simulink subsystem "Shooter_Arm_Controls"  (R2023b)
settings: Solver=VariableStepAuto  StartTime=0.0  StopTime=10.0  RelTol=1e-3
undefined symbols (not defined in the file): Back_AA_Bot_Max_Ext, Back_AA_Bot_Min_Ext, Back_AA_length, Back_AA_spacing, Back_AA_Top_Max_Ext, Back_AA_Top_Min_Ext, Front_AA_length, Front_AA_Max_Ext, Front_AA_Min_Ext, Front_AA_spacing, l_1, l_10, l_11, l_2, l_3, l_4, l_5, l_6, l_7, l_8, l_9, Speaker_Angle_out, Speaker_Distance_in, Speaker_Distance_Offset, Speaker_Gap_out, Speaker_Height_out, TEST_Speaker_Angle, TEST_Speaker_Gap, TEST_Speaker_Height
libraries: Controls_Components_lib x5, simulink x4, simulink_need_slupdate x3
settings Model: Creator=ander  LastModifiedBy=ander

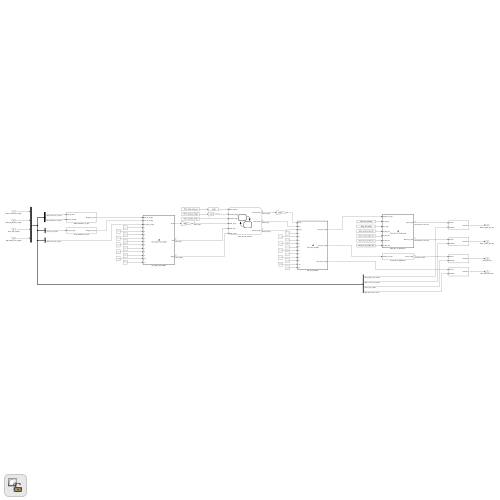
[thumbnail: Simulink's stored preview of the top-level diagram]
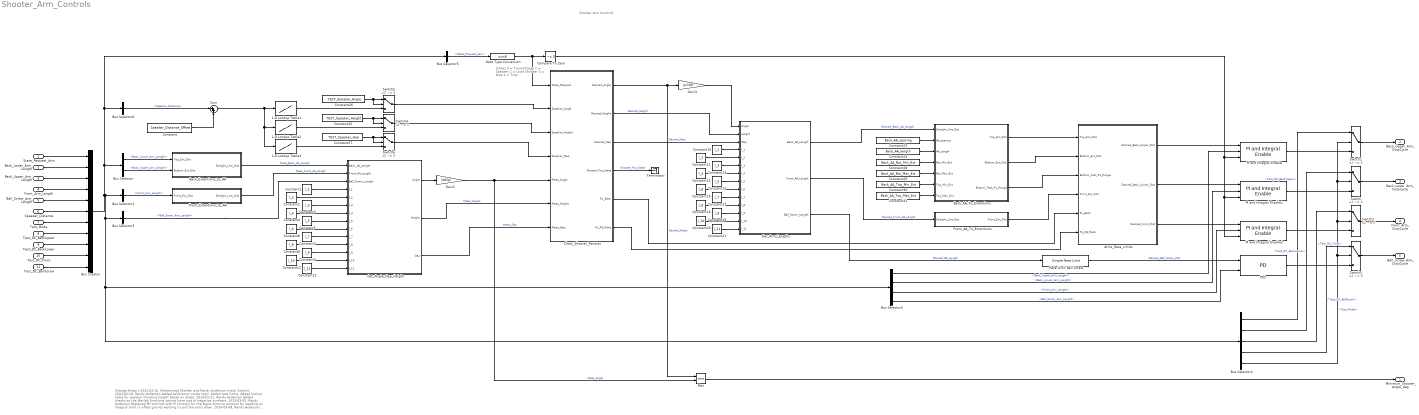
== system Shooter_Arm_Controls ==
  note: Shooter Arm Controls
  note: Change History
      | 2024-02-15, Mohammad Kherfan and Randy Anderson
      | Initial Commit
      | 2024-02-18, Randy Anderson
      | Added calibration mode logic.
      | Added rate limits.
      | Added lookup table for speaker shooting height based on angle.
      | 2024-02-21, Randy Anderson
      | Added checks so the Matlab functions cannot have sqrt of negative numbers.
      | 2024-03-05, Randy Anderson
      | Replaced PD controls with PI controls for the Argos Arms to account for needing an
      | integral term to offset gravity wanting to pull the arms down.
      | 2024-03-08, Randy Anderson
      | Removed calibration mode logic
      | Added test mode duty cycle inputs
      | 2024-03-09, Janelyn Anderson and Randy Anderson
      | Modified the Matlab function to "Back_AA_To_Extentions"
  note: States
      | 0 = Travel/Stage
      | 1 = Speaker
      | 2 = Load Shooter
      | 3 = Amp
      | 4 = Trap
  State_Request_Arm : Inport
  Back_Lower_Arm_Length : Inport  Port=2
  Back_Upper_Arm_Length : Inport  Port=3
  Front_Arm_Length : Inport  Port=4
  Ball_Screw_Arm_Length : Inport  Port=5
  Speaker_Distance : Inport  Port=6
  Test_Mode : Inport  Port=7
  Test_DC_BackUpper : Inport  Port=8
  Test_DC_BackLower : Inport  Port=9
  Test_DC_Front : Inport  Port=10
  Test_DC_BallScrew : Inport  Port=11
  1-D Lookup Table1 : Lookup_n-D  NumberOfTableDimensions=1  BreakpointsForDimension1=Speaker_Distance_in  Table=Speaker_Angle_out  ExtrapMethod=Clip  InternalRulePriority=Speed  RndMeth=Simplest
  1-D Lookup Table2 : Lookup_n-D  NumberOfTableDimensions=1  BreakpointsForDimension1=Speaker_Distance_in  Table=Speaker_Height_out  ExtrapMethod=Clip  InternalRulePriority=Speed  RndMeth=Simplest
  1-D Lookup Table3 : Lookup_n-D  NumberOfTableDimensions=1  BreakpointsForDimension1=Speaker_Distance_in  Table=Speaker_Gap_out  ExtrapMethod=Clip  InternalRulePriority=Speed  RndMeth=Simplest
  Arms_Rate_Limits : Subsystem
  Back_AA_To_Extentions : MATLAB Function  TreatAsAtomicUnit=on
  Back_Extentions_to_AA : Subsystem
  Bus Creator : BusCreator  Inputs=11
  Bus Selector : BusSelector  OutputSignals=Back_Lower_Arm_Length,Back_Upper_Arm_Length
  Bus Selector1 : BusSelector  OutputSignals=Front_Arm_Length
  Bus Selector2 : BusSelector  OutputSignals=Back_Upper_Arm_Length,Back_Lower_Arm_Length,Front_Arm_Length,Ball_Screw_Arm_Length
  Bus Selector3 : BusSelector  OutputSignals=Ball_Screw_Arm_Length
  Bus Selector4 : BusSelector  OutputSignals=Test_DC_BackUpper,Test_DC_BackLower,Test_DC_Front,Test_DC_BallScrew,Test_Mode
  Bus Selector5 : BusSelector  OutputSignals=State_Request_Arm
  Bus Selector6 : BusSelector  OutputSignals=Speaker_Distance
  Chart_Shooter_Position : Stateflow chart  TreatAsAtomicUnit=on
  Compare To Zero : simulink/Logic and Bit Operations/Compare To Zero  relop=~=  OutDataTypeStr=boolean
  Constant : Constant  Value=Speaker_Distance_Offset
  Constant1 : Constant  Value=l_1
  Constant10 : Constant  Value=l_1
  Constant11 : Constant  Value=l_2
  Constant12 : Constant  Value=l_10
  Constant13 : Constant  Value=l_3
  Constant14 : Constant  Value=l_4
  Constant15 : Constant  Value=l_5
  Constant16 : Constant  Value=l_6
  Constant17 : Constant  Value=l_7
  Constant18 : Constant  Value=l_8
  Constant19 : Constant  Value=l_9
  Constant2 : Constant  Value=l_2
  Constant20 : Constant  Value=l_10
  Constant21 : Constant  Value=l_11
  Constant22 : Constant  Value=l_11
  Constant23 : Constant  Value=Back_AA_spacing
  Constant24 : Constant  Value=Back_AA_length
  Constant25 : Constant  Value=TEST_Speaker_Height
  Constant26 : Constant  Value=TEST_Speaker_Angle
  Constant27 : Constant  Value=TEST_Speaker_Gap
  Constant28 : Constant  Value=Back_AA_Bot_Min_Ext
  Constant29 : Constant  Value=Back_AA_Bot_Max_Ext
  Constant3 : Constant  Value=l_3
  Constant30 : Constant  Value=Back_AA_Top_Min_Ext
  Constant31 : Constant  Value=Back_AA_Top_Max_Ext
  Constant4 : Constant  Value=l_4
  Constant5 : Constant  Value=l_5
  Constant6 : Constant  Value=l_6
  Constant7 : Constant  Value=l_7
  Constant8 : Constant  Value=l_8
  Constant9 : Constant  Value=l_9
  Data Type Conversion : DataTypeConversion  OutDataTypeStr=uint8  SaturateOnIntegerOverflow=off  RndMeth=Floor
  Front_AA_To_Extentions : Subsystem
  Front_Extentions_to_AA : Subsystem
  Gain2 : Gain  Gain=180/pi
  Gain3 : Gain  Gain=pi/180
  Get_Angle_Gap_Height : MATLAB Function  TreatAsAtomicUnit=on
  Get_Arm_Lengths : MATLAB Function  TreatAsAtomicUnit=on
  Max : MinMax  Inputs=2
  PD3 : Controls_Components_lib/PD  Gain_P=BS_Prop_Gain  Gain_D=BS_Deriv_Gain  FilterCoeff_D=BS_Deriv_FC  Limit_D_Upper=BS_Deriv_UL  Limit_D_Lower=BS_Deriv_LL  Limit_T_Upper=BS_TC_UL  Limit_T_Lower=BS_TC_LL
  PI and Integral Enable : Controls_Components_lib/PI and Integral Enable  Gain_P=AA_Prop_Gain  Gain_I=AA_Integral_Gain  Integral_IC=AA_Integral_IC  Limit_I_Upper=AA_Integral_UL  Limit_I_Lower=AA_Integral_LL  Limit_T_Upper=AA_TC_UL  Limit_T_Lower=AA_TC_LL
  PI and Integral Enable1 : Controls_Components_lib/PI and Integral Enable  Gain_P=AA_Prop_Gain  Gain_I=AA_Integral_Gain  Integral_IC=AA_Integral_IC  Limit_I_Upper=AA_Integral_UL  Limit_I_Lower=AA_Integral_LL  Limit_T_Upper=AA_TC_UL  Limit_T_Lower=AA_TC_LL
  PI and Integral Enable2 : Controls_Components_lib/PI and Integral Enable  Gain_P=AA_Prop_Gain  Gain_I=AA_Integral_Gain  Integral_IC=AA_Integral_IC  Limit_I_Upper=AA_Integral_UL  Limit_I_Lower=AA_Integral_LL  Limit_T_Upper=AA_TC_UL  Limit_T_Lower=AA_TC_LL
  Rate Limit Ball Screw : Controls_Components_lib/Simple Rate Limit  Rate_Limit_Inc=BS_Position_Inc_RL  Rate_Limit_Dec=BS_Position_Dec_RL
  Sum : Sum  Inputs=|++
  Switch{,1..6} (7 alike) : Switch  Criteria=u2 ~= 0  SaturateOnIntegerOverflow=off  InputSameDT=off
  Terminator : Terminator
  Minimum_Shooter_Angle_deg : Outport
  Back_Upper_Arm_DutyCycle : Outport  Port=2
  Back_Lower_Arm_DutyCycle : Outport  Port=3
  Front_Arm_DutyCycle : Outport  Port=4
  Ball_Screw_Arm_DutyCycle : Outport  Port=5
  wires:
  Constant12/1 -> Get_Angle_Gap_Height/13(l_10)
  Constant6/1 -> Get_Angle_Gap_Height/9(l_6)
  Constant2/1 -> Get_Angle_Gap_Height/5(l_2)
  Constant7/1 -> Get_Angle_Gap_Height/10(l_7)
  Constant8/1 -> Get_Angle_Gap_Height/11(l_8)
  Constant22/1 -> Get_Angle_Gap_Height/14(l_11)
  Constant4/1 -> Get_Angle_Gap_Height/7(l_4)
  Constant9/1 -> Get_Angle_Gap_Height/12(l_9)
  Constant5/1 -> Get_Angle_Gap_Height/8(l_5)
  Constant3/1 -> Get_Angle_Gap_Height/6(l_3)
  Constant1/1 -> Get_Angle_Gap_Height/4(l_1)
  Back_Extentions_to_AA/1(Straight_Line_Dist) -> Get_Angle_Gap_Height/1(Back_AA_Length)  "Meas_Back_AA_Length"
  Front_Extentions_to_AA/1(Straight_Line_Dist) -> Get_Angle_Gap_Height/2(Front_AA_Length)  "Meas_Front_AA_Length"
  Get_Angle_Gap_Height/1(Angle) -> Gain2/1
  Get_Angle_Gap_Height/3(Gap) -> Chart_Shooter_Position/7(Meas_Gap)  "Meas_Gap"
  Get_Angle_Gap_Height/2(Height) -> Chart_Shooter_Position/6(Meas_Height)  "Meas_Height"
  Constant20/1 -> Get_Arm_Lengths/13(l_10)
  Constant18/1 -> Get_Arm_Lengths/11(l_8)
  Constant14/1 -> Get_Arm_Lengths/7(l_4)
  Constant10/1 -> Get_Arm_Lengths/4(l_1)
  Constant21/1 -> Get_Arm_Lengths/14(l_11)
  Constant15/1 -> Get_Arm_Lengths/8(l_5)
  Constant16/1 -> Get_Arm_Lengths/9(l_6)
  Constant13/1 -> Get_Arm_Lengths/6(l_3)
  Constant17/1 -> Get_Arm_Lengths/10(l_7)
  Constant19/1 -> Get_Arm_Lengths/12(l_9)
  Constant11/1 -> Get_Arm_Lengths/5(l_2)
  Chart_Shooter_Position/3(Desired_Gap) -> Get_Arm_Lengths/3(Gap)  "Desired_Gap"
  Chart_Shooter_Position/2(Desired_Height) -> Get_Arm_Lengths/2(Height)  "Desired_Height"
  Chart_Shooter_Position/1(Desired_Angle) -> Gain3/1, Max/1  "Desired_Angle"
  Constant24/1 -> Back_AA_To_Extentions/3(AA_Length)
  Constant31/1 -> Back_AA_To_Extentions/7(Top_Max_Ext)
  Constant29/1 -> Back_AA_To_Extentions/5(Bot_Max_Ext)
  Constant30/1 -> Back_AA_To_Extentions/6(Top_Min_Ext)
  Constant28/1 -> Back_AA_To_Extentions/4(Bot_Min_Ext)
  Constant23/1 -> Back_AA_To_Extentions/2(AA_spacing)
  Get_Arm_Lengths/1(Back_AA_Length) -> Back_AA_To_Extentions/1(Straight_Line_Dist)  "Desired_Back_AA_Length"
  Get_Arm_Lengths/2(Front_AA_Length) -> Front_AA_To_Extentions/1(Straight_Line_Dist)  "Desired_Front_AA_Length"
  Get_Arm_Lengths/3(Ball_Screw_Length) -> Rate Limit Ball Screw/1  "Desired_BS_Length"
  Back_Lower_Arm_Length/1 -> Bus Creator/2
  Back_Upper_Arm_Length/1 -> Bus Creator/3
  Front_Arm_Length/1 -> Bus Creator/4
  Ball_Screw_Arm_Length/1 -> Bus Creator/5
  Bus Creator/1 -> Bus Selector1/1, Bus Selector3/1, Bus Selector2/1, Bus Selector4/1, Bus Selector/1, Bus Selector6/1, Bus Selector5/1
  Bus Selector/1 -> Back_Extentions_to_AA/1(Top_Ext_Dist)  "<Back_Lower_Arm_Length>"
  Bus Selector/2 -> Back_Extentions_to_AA/2(Bottom_Ext_Dist)  "<Back_Upper_Arm_Length>"
  Bus Selector1/1 -> Front_Extentions_to_AA/1(Front_Ext_Dist)  "<Front_Arm_Length>"
  Bus Selector2/4 -> PD3/2  "<Ball_Screw_Arm_Length>"
  Bus Selector2/3 -> PI and Integral Enable2/2  "<Front_Arm_Length>"
  Bus Selector2/1 -> PI and Integral Enable/2  "<Back_Upper_Arm_Length>"
  Bus Selector2/2 -> PI and Integral Enable1/2  "<Back_Lower_Arm_Length>"
  Bus Selector3/1 -> Get_Angle_Gap_Height/3(Ball_Screw_Length)  "<Ball_Screw_Arm_Length>"
  Gain2/1 -> Chart_Shooter_Position/5(Meas_Angle), Max/2  "Meas_Angle"
  Gain3/1 -> Get_Arm_Lengths/1(Angle)
  Data Type Conversion/1 -> Chart_Shooter_Position/1(State_Request), Compare To Zero/1
  Test_Mode/1 -> Bus Creator/7
  PI and Integral Enable1/1 -> Switch/3
  PI and Integral Enable/1 -> Switch1/3
  PI and Integral Enable2/1 -> Switch2/3
  PD3/1 -> Switch3/3
  Switch1/1 -> Back_Upper_Arm_DutyCycle/1
  Switch/1 -> Back_Lower_Arm_DutyCycle/1
  Switch2/1 -> Front_Arm_DutyCycle/1
  Switch3/1 -> Ball_Screw_Arm_DutyCycle/1
  Test_DC_Front/1 -> Bus Creator/10
  Test_DC_BallScrew/1 -> Bus Creator/11
  Rate Limit Ball Screw/1 -> PD3/1  "Desired_Ball_Screw_Dist"
  Switch5/1 -> Chart_Shooter_Position/2(Speaker_Angle)
  State_Request_Arm/1 -> Bus Creator/1
  Bus Selector5/1 -> Data Type Conversion/1  "<State_Request_Arm>"
  Compare To Zero/1 -> PI and Integral Enable/3, PI and Integral Enable1/3, PI and Integral Enable2/3
  Chart_Shooter_Position/4(Shooter_Pos_State) -> Terminator/1  "Shooter_Pos_State"
  Test_DC_BackUpper/1 -> Bus Creator/8
  Test_DC_BackLower/1 -> Bus Creator/9
  Bus Selector4/1 -> Switch1/1  "<Test_DC_BackUpper>"
  Bus Selector4/2 -> Switch/1  "<Test_DC_BackLower>"
  Bus Selector4/3 -> Switch2/1  "<Test_DC_Front>"
  Bus Selector4/4 -> Switch3/1  "<Test_DC_BallScrew>"
  Bus Selector4/5 -> Switch3/2, Switch2/2, Switch/2, Switch1/2  "<Test_Mode>"
  Constant26/1 -> Switch5/2, Switch5/1
  Speaker_Distance/1 -> Bus Creator/6
  1-D Lookup Table1/1 -> Switch5/3
  Max/1 -> Minimum_Shooter_Angle_deg/1
  1-D Lookup Table2/1 -> Switch4/3
  Constant25/1 -> Switch4/1, Switch4/2
  Switch4/1 -> Chart_Shooter_Position/3(Speaker_Height)
  Constant27/1 -> Switch6/2, Switch6/1
  1-D Lookup Table3/1 -> Switch6/3
  Switch6/1 -> Chart_Shooter_Position/4(Speaker_Gap)
  Back_AA_To_Extentions/1(Top_Ext_Dist) -> Arms_Rate_Limits/1(Top_Ext_Dist)
  Back_AA_To_Extentions/2(Bottom_Ext_Dist) -> Arms_Rate_Limits/2(Bottom_Ext_Dist)
  Back_AA_To_Extentions/3(Bottom_Fast_RL_Range) -> Arms_Rate_Limits/3(Bottom_Fast_RL_Range)
  Front_AA_To_Extentions/1(Front_Ext_Dist) -> Arms_Rate_Limits/4(Front_Ext_Dist)
  Arms_Rate_Limits/1(Desired_Back_Upper_Dist) -> PI and Integral Enable/1
  Arms_Rate_Limits/2(Desired_Back_Lower_Dist) -> PI and Integral Enable1/1
  Arms_Rate_Limits/3(Desired_Front_Dist) -> PI and Integral Enable2/1
  Chart_Shooter_Position/5(RL_Back) -> Arms_Rate_Limits/5(RL_Back)
  Chart_Shooter_Position/6(RL_FB_Ratio) -> Arms_Rate_Limits/6(RL_FB_Ratio)
  Bus Selector6/1 -> Sum/1  "<Speaker_Distance>"
  Sum/1 -> 1-D Lookup Table1/1, 1-D Lookup Table3/1, 1-D Lookup Table2/1
  Constant/1 -> Sum/2

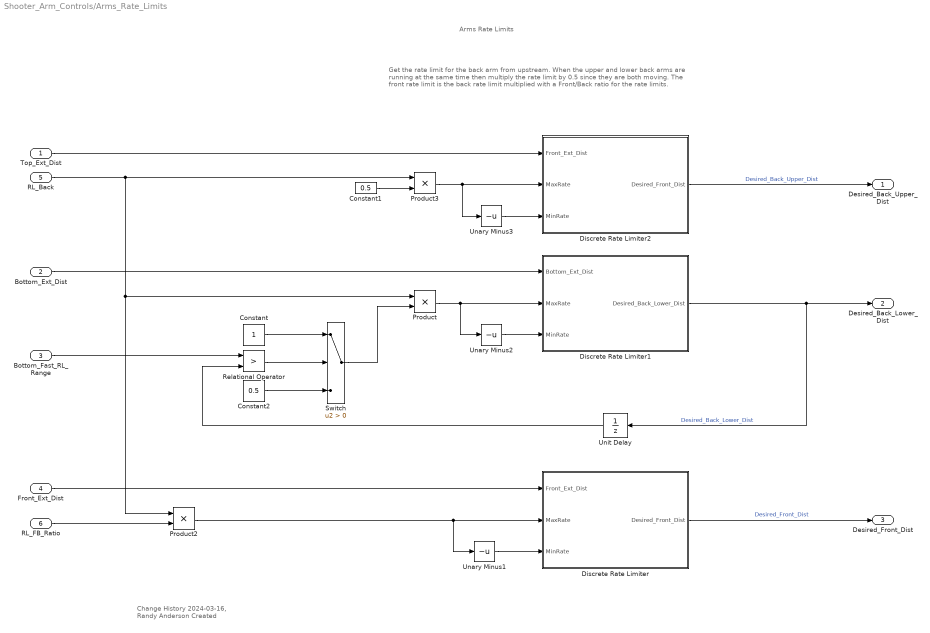
== system Shooter_Arm_Controls/Arms_Rate_Limits ==
  note: Change History
      | 2024-03-16, Randy Anderson
      | Created
  note: Arms Rate Limits
  note: Get the rate limit for the back arm from upstream.  When the upper and lower back arms are running at the same time then multiply the rate limit by 0.5 since they are both moving.
      |
      | The front rate limit is the back rate limit multiplied with a Front/Back ratio for the rate limits.
  Top_Ext_Dist : Inport
  Bottom_Ext_Dist : Inport  Port=2
  Bottom_Fast_RL_Range : Inport  Port=3
  Front_Ext_Dist : Inport  Port=4
  RL_Back : Inport  Port=5
  RL_FB_Ratio : Inport  Port=6
  Constant : Constant
  Constant1 : Constant  Value=0.5
  Constant2 : Constant  Value=0.5
  Discrete Rate Limiter : Subsystem
  Discrete Rate Limiter1 : Subsystem
  Discrete Rate Limiter2 : Subsystem
  Product : Product
  Product2 : Product
  Product3 : Product
  Relational Operator : RelationalOperator  Operator=>  OutDataTypeStr=boolean  RndMeth=Simplest  InputSameDT=off
  Switch : Switch  Criteria=u2 > Threshold  SaturateOnIntegerOverflow=off  InputSameDT=off
  Unary Minus1 : UnaryMinus
  Unary Minus2 : UnaryMinus
  Unary Minus3 : UnaryMinus
  Unit Delay : UnitDelay  SampleTime=-1  HasFrameUpgradeWarning=on
  Desired_Back_Upper_Dist : Outport
  Desired_Back_Lower_Dist : Outport  Port=2
  Desired_Front_Dist : Outport  Port=3
  wires:
  Unary Minus3/1 -> Discrete Rate Limiter2/3(MinRate)
  Unary Minus2/1 -> Discrete Rate Limiter1/3(MinRate)
  Unary Minus1/1 -> Discrete Rate Limiter/3(MinRate)
  Product2/1 -> Discrete Rate Limiter/2(MaxRate), Unary Minus1/1
  Constant1/1 -> Product3/2
  Product3/1 -> Unary Minus3/1, Discrete Rate Limiter2/2(MaxRate)
  Top_Ext_Dist/1 -> Discrete Rate Limiter2/1(Front_Ext_Dist)
  Bottom_Ext_Dist/1 -> Discrete Rate Limiter1/1(Bottom_Ext_Dist)
  RL_FB_Ratio/1 -> Product2/2
  RL_Back/1 -> Product3/1, Product2/1, Product/1
  Front_Ext_Dist/1 -> Discrete Rate Limiter/1(Front_Ext_Dist)
  Bottom_Fast_RL_Range/1 -> Relational Operator/1
  Constant/1 -> Switch/1
  Switch/1 -> Product/2
  Product/1 -> Unary Minus2/1, Discrete Rate Limiter1/2(MaxRate)
  Constant2/1 -> Switch/3
  Relational Operator/1 -> Switch/2
  Unit Delay/1 -> Relational Operator/2
  Discrete Rate Limiter1/1(Desired_Back_Lower_Dist) -> Desired_Back_Lower_Dist/1, Unit Delay/1  "Desired_Back_Lower_Dist"
  Discrete Rate Limiter2/1(Desired_Front_Dist) -> Desired_Back_Upper_Dist/1  "Desired_Back_Upper_Dist"
  Discrete Rate Limiter/1(Desired_Front_Dist) -> Desired_Front_Dist/1  "Desired_Front_Dist"

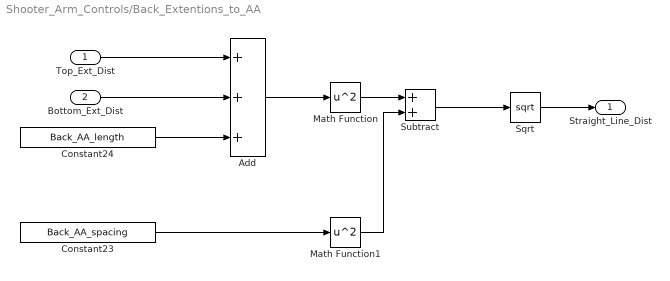
== system Shooter_Arm_Controls/Back_Extentions_to_AA ==
  Top_Ext_Dist : Inport
  Bottom_Ext_Dist : Inport  Port=2
  Add : Sum  Inputs=+++
  Constant23 : Constant  Value=Back_AA_spacing
  Constant24 : Constant  Value=Back_AA_length
  Math Function : Math  Operator=square
  Math Function1 : Math  Operator=square
  Sqrt : Sqrt
  Subtract : Sum  Inputs=2
  Straight_Line_Dist : Outport
  wires:
  Sqrt/1 -> Straight_Line_Dist/1
  Subtract/1 -> Sqrt/1
  Math Function1/1 -> Subtract/2
  Math Function/1 -> Subtract/1
  Constant23/1 -> Math Function1/1
  Add/1 -> Math Function/1
  Constant24/1 -> Add/3
  Bottom_Ext_Dist/1 -> Add/2
  Top_Ext_Dist/1 -> Add/1

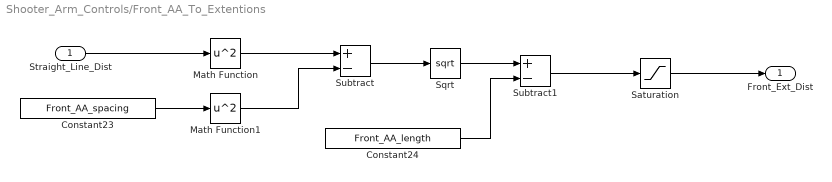
== system Shooter_Arm_Controls/Front_AA_To_Extentions ==
  Straight_Line_Dist : Inport
  Constant23 : Constant  Value=Front_AA_spacing
  Constant24 : Constant  Value=Front_AA_length
  Math Function : Math  Operator=square
  Math Function1 : Math  Operator=square
  Saturation : Saturate  UpperLimit=Front_AA_Max_Ext  LowerLimit=Front_AA_Min_Ext
  Sqrt : Sqrt
  Subtract : Sum  Inputs=+-
  Subtract1 : Sum  Inputs=+-
  Front_Ext_Dist : Outport
  wires:
  Saturation/1 -> Front_Ext_Dist/1
  Subtract1/1 -> Saturation/1
  Constant24/1 -> Subtract1/2
  Sqrt/1 -> Subtract1/1
  Straight_Line_Dist/1 -> Math Function/1
  Constant23/1 -> Math Function1/1
  Math Function/1 -> Subtract/1
  Math Function1/1 -> Subtract/2
  Subtract/1 -> Sqrt/1

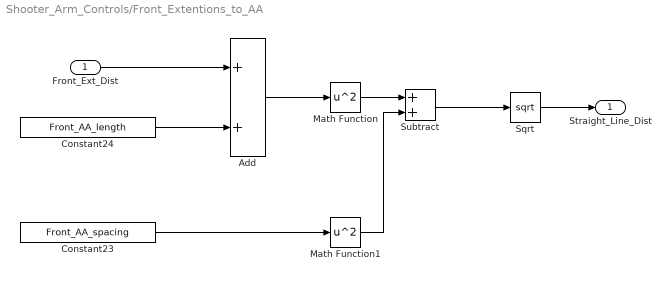
== system Shooter_Arm_Controls/Front_Extentions_to_AA ==
  Front_Ext_Dist : Inport
  Add : Sum  Inputs=2
  Constant23 : Constant  Value=Front_AA_spacing
  Constant24 : Constant  Value=Front_AA_length
  Math Function : Math  Operator=square
  Math Function1 : Math  Operator=square
  Sqrt : Sqrt
  Subtract : Sum  Inputs=2
  Straight_Line_Dist : Outport
  wires:
  Math Function1/1 -> Subtract/2
  Math Function/1 -> Subtract/1
  Constant23/1 -> Math Function1/1
  Constant24/1 -> Add/2
  Add/1 -> Math Function/1
  Sqrt/1 -> Straight_Line_Dist/1
  Front_Ext_Dist/1 -> Add/1
  Subtract/1 -> Sqrt/1

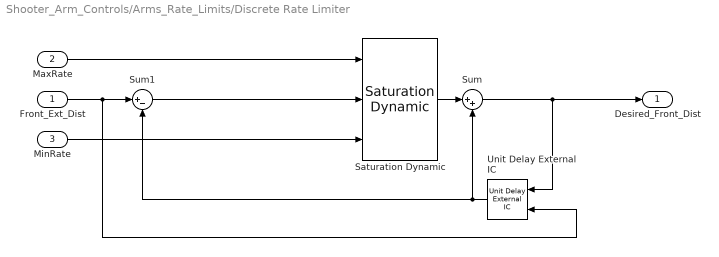
== system Shooter_Arm_Controls/Arms_Rate_Limits/Discrete Rate Limiter ==
  Front_Ext_Dist : Inport
  MaxRate : Inport  Port=2
  MinRate : Inport  Port=3
  Saturation Dynamic : simulink/Discontinuities/Saturation Dynamic  OutMin=[]  OutMax=[]  OutDataTypeStr=Inherit: Same as second input  OutDataType=fixdt(1, 16)  OutScaling=2^-10  DoSatur=off
  Sum : Sum  Inputs=|++  OutDataTypeStr=Inherit: Inherit via back propagation
  Sum1 : Sum  Inputs=|+-  OutDataTypeStr=Inherit: Inherit via back propagation  SaturateOnIntegerOverflow=on
  Unit Delay External IC : simulink_need_slupdate/Unit Delay External IC  tsamp=-1
  Desired_Front_Dist : Outport
  wires:
  Front_Ext_Dist/1 -> Sum1/1, Unit Delay External IC/2
  Unit Delay External IC/1 -> Sum/2, Sum1/2
  Sum1/1 -> Saturation Dynamic/2
  Saturation Dynamic/1 -> Sum/1
  MaxRate/1 -> Saturation Dynamic/1
  MinRate/1 -> Saturation Dynamic/3
  Sum/1 -> Unit Delay External IC/1, Desired_Front_Dist/1

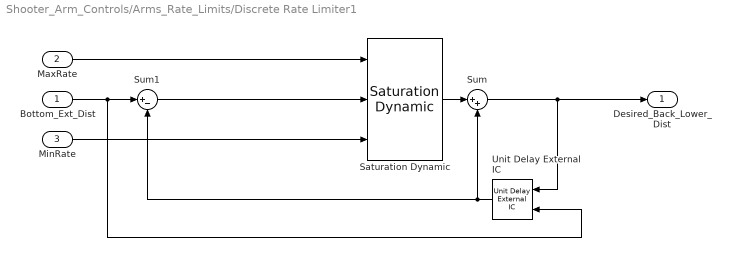
== system Shooter_Arm_Controls/Arms_Rate_Limits/Discrete Rate Limiter1 ==
  Bottom_Ext_Dist : Inport
  MaxRate : Inport  Port=2
  MinRate : Inport  Port=3
  Saturation Dynamic : simulink/Discontinuities/Saturation Dynamic  OutMin=[]  OutMax=[]  OutDataTypeStr=Inherit: Same as second input  OutDataType=fixdt(1, 16)  OutScaling=2^-10  DoSatur=off
  Sum : Sum  Inputs=|++  OutDataTypeStr=Inherit: Inherit via back propagation
  Sum1 : Sum  Inputs=|+-  OutDataTypeStr=Inherit: Inherit via back propagation  SaturateOnIntegerOverflow=on
  Unit Delay External IC : simulink_need_slupdate/Unit Delay External IC  tsamp=-1
  Desired_Back_Lower_Dist : Outport
  wires:
  Bottom_Ext_Dist/1 -> Sum1/1, Unit Delay External IC/2
  Unit Delay External IC/1 -> Sum/2, Sum1/2
  Sum1/1 -> Saturation Dynamic/2
  Saturation Dynamic/1 -> Sum/1
  MaxRate/1 -> Saturation Dynamic/1
  MinRate/1 -> Saturation Dynamic/3
  Sum/1 -> Unit Delay External IC/1, Desired_Back_Lower_Dist/1

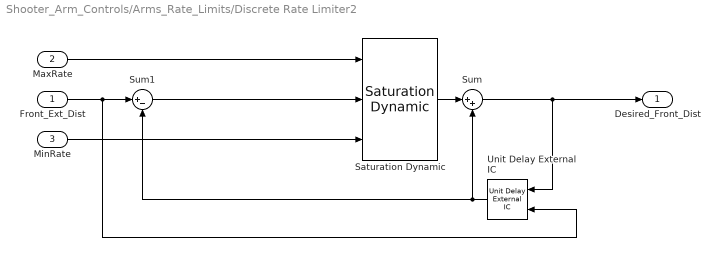
== system Shooter_Arm_Controls/Arms_Rate_Limits/Discrete Rate Limiter2 ==
  Front_Ext_Dist : Inport
  MaxRate : Inport  Port=2
  MinRate : Inport  Port=3
  Saturation Dynamic : simulink/Discontinuities/Saturation Dynamic  OutMin=[]  OutMax=[]  OutDataTypeStr=Inherit: Same as second input  OutDataType=fixdt(1, 16)  OutScaling=2^-10  DoSatur=off
  Sum : Sum  Inputs=|++  OutDataTypeStr=Inherit: Inherit via back propagation
  Sum1 : Sum  Inputs=|+-  OutDataTypeStr=Inherit: Inherit via back propagation  SaturateOnIntegerOverflow=on
  Unit Delay External IC : simulink_need_slupdate/Unit Delay External IC  tsamp=-1
  Desired_Front_Dist : Outport
  wires:
  Sum/1 -> Desired_Front_Dist/1, Unit Delay External IC/1
  MinRate/1 -> Saturation Dynamic/3
  MaxRate/1 -> Saturation Dynamic/1
  Saturation Dynamic/1 -> Sum/1
  Sum1/1 -> Saturation Dynamic/2
  Unit Delay External IC/1 -> Sum1/2, Sum/2
  Front_Ext_Dist/1 -> Unit Delay External IC/2, Sum1/1

== stateflow chart Shooter_Arm_Controls/Chart_Shooter_Position ==
  state Stage
    en: Shooter_Pos_State = 0;
    Desired_Angle = Stage_Angle;
    Desired_Height = Stage_Height;
    Desired_Gap = Stage_Gap;
  state Stage_to_Speaker
    en: Shooter_Pos_State = 1;
    Desired_Height = Speaker_Height;
  state Speaker
    en: Shooter_Pos_State = 2;
    Desired_Angle = Speaker_Angle;
    Desired_Height = Speaker_Height;
    Desired_Gap = Speaker_Gap;
    du:
    Desired_Angle = Speaker_Angle;
    Desired_Height = Speaker_Height;
    Desired_Gap = Speaker_Gap;
  state Speaker_to_Stage
    en: Shooter_Pos_State = 3;
    Desired_Angle = Stage_Angle;
    Desired_Gap = Stage_Gap;
  state Amp
    en: Shooter_Pos_State = 4;
    Desired_Angle = Amp_Angle;
    Desired_Height = Amp_Height;
    Desired_Gap = Amp_Gap;
  state LoadShooter
    en: Shooter_Pos_State = 5;
    Desired_Angle = LoadShooter_Angle;
    Desired_Height = LoadShooter_Height;
    Desired_Gap = LoadShooter_Gap;
  state Trap
    en: Shooter_Pos_State = 6;
    Desired_Angle = Trap_Angle;
    Desired_Height = Trap_Height;
    Desired_Gap = Trap_Gap;
  (default) -> Stage
  Stage_to_Speaker -> Speaker : [Meas_Height < (Speaker_Height + Tol_Height) && ...
      | Meas_Height > (Speaker_Height - Tol_Height)]
      | {RL_Back = RL_Back_Speaker_Partial_to_Speaker_Final;
      |  RL_FB_Ratio = RL_FB_Ratio_Speaker_Final;}
  Stage -> Stage_to_Speaker [order 1] : [State_Request == State_Speaker]
      | {RL_Back = RL_Back_Stage_to_Speaker_Partial; ...
      |  RL_FB_Ratio = RL_FB_Ratio_Speaker_Partial;}
  Speaker -> Speaker_to_Stage : [State_Request == State_Stage]
      | {RL_Back = RL_Back_Speaker_Final_to_Speaker_Partial; ...
      |  RL_FB_Ratio =  RL_FB_Ratio_Speaker_Final;}
  Speaker_to_Stage -> Stage : [Meas_Angle < (Stage_Angle + Tol_Angle) && ...
      | Meas_Angle > (Stage_Angle - Tol_Angle) && ...
      | Meas_Gap < (Stage_Gap + Tol_Gap) && ...
      | Meas_Gap > (Stage_Gap - Tol_Gap)]
      | {RL_Back = RL_Back_Speaker_Partial_to_Stage; ...
      |  RL_FB_Ratio = RL_FB_Ratio_Speaker_Partial;}
  Stage -> Amp [order 4] : [State_Request == State_Amp]
      | {RL_Back = RL_Back_Stage_to_Amp; ...
      |  RL_FB_Ratio = RL_FB_Ratio_Stage_Amp;}
  Amp -> Stage : [State_Request == State_Stage]
      | {RL_Back = RL_Back_Amp_to_Stage; ...
      |  RL_FB_Ratio = RL_FB_Ratio_Stage_Amp;}
  Stage -> LoadShooter [order 2] : [State_Request == State_LoadShooter]
      | {RL_Back = RL_Back_Stage_to_Load; ...
      |  RL_FB_Ratio = RL_FB_Ratio_Stage_Load;}
  LoadShooter -> Amp [order 2] : [State_Request == State_Amp]
      | {RL_Back = RL_Back_Load_to_Amp; ...
      |  RL_FB_Ratio = RL_FB_Ratio_Load_Amp;}
  LoadShooter -> Stage [order 1] : [State_Request == State_Stage]
      | {RL_Back = RL_Back_Load_to_Stage; ...
      |  RL_FB_Ratio = RL_FB_Ratio_Stage_Load;}
  Stage -> Trap [order 3] : [State_Request == State_Trap]
      | {RL_Back = RL_Back_Stage_to_Trap; ...
      |  RL_FB_Ratio = RL_FB_Ratio_Stage_Trap;}
  Trap -> Stage : [State_Request == State_Stage]
      | {RL_Back = RL_Back_Trap_to_Stage; ...
      |  RL_FB_Ratio = RL_FB_Ratio_Stage_Trap;}
  data: State_Request input uint8 size=1; Speaker_Angle input double size=1; Desired_Angle output double size=1; Desired_Height output double size=1; Desired_Gap output double size=1; Speaker_Height input double size=1; Speaker_Gap input double size=1; Meas_Angle input double size=1; Meas_Height input double size=1; Meas_Gap input double size=1; LoadShooter_Gap parameter double size=1; Amp_Gap parameter double size=1; Trap_Gap parameter double size=1; LoadShooter_Height parameter double size=1; Amp_Angle parameter double size=1; LoadShooter_Angle parameter double size=1; Stage_Height parameter double size=1; Trap_Angle parameter double size=1; Trap_Height parameter double size=1; Stage_Angle parameter double size=1; Amp_Height parameter double size=1; Stage_Gap parameter double size=1; State_Trap constant uint8 =4; State_LoadShooter constant uint8 =2; State_Stage constant uint8 =0; State_Amp constant uint8 =3; State_Speaker constant uint8 =1; Tol_Height parameter double size=1; Tol_Gap parameter double size=1; Tol_Angle parameter double size=1; Shooter_Pos_State output double; RL_Back_Speaker_Final_to_Speaker_Partial parameter; RL_FB_Ratio_Speaker_Final parameter; RL_Back_Speaker_Partial_to_Speaker_Final parameter; RL_Back_Stage_to_Speaker_Partial parameter; RL_FB_Ratio_Speaker_Partial parameter; RL_Back_Speaker_Partial_to_Stage parameter; RL_FB_Ratio_Stage_Amp parameter; RL_Back_Stage_to_Load parameter; RL_Back_Amp_to_Stage parameter; RL_Back_Load_to_Amp parameter; RL_FB_Ratio_Load_Amp parameter; RL_FB_Ratio_Stage_Load parameter; RL_Back_Trap_to_Stage parameter; RL_Back_Stage_to_Trap parameter; RL_Back_Stage_to_Amp parameter; RL_FB_Ratio_Stage_Trap parameter; RL_Back_Load_to_Stage parameter; RL_Back output; RL_FB_Ratio output

== matlab function Shooter_Arm_Controls/Get_Angle_Gap_Height ==
  data: Angle output; Height output; Gap output; Back_AA_Length input; Front_AA_Length input; Ball_Screw_Length input; l_1 input; l_2 input; l_3 input; l_4 input; l_5 input; l_6 input; l_7 input; l_8 input; l_9 input; l_10 input; l_11 input
function [Angle, Height, Gap] = Get_Angle_Gap_Height(Back_AA_Length,Front_AA_Length,Ball_Screw_Length,l_1,l_2,l_3,l_4,l_5,l_6,l_7,l_8,l_9,l_10,l_11)

% Kinematic lengths
% l_1: vertical offset of back Argos Arm
% l_2: vertical offset of Ball Screw
% l_3: horizontal length from back argos arm to Ball Screw
% l_4: horizontal length from ball screw to front Argos Arm
% l_5: length from pivot of front argos arm to pivot of ball screw on that arm
% l_6: horizontal offset from the end of gap to Back Argos Arm pivot on shooter
% l_7: vertical offset from the end of gap to Back Argos Arm pivot on shooter
% l_8: horizontal offset from back argos arm to Front Argos Arm pivot on shooter
% l_9: vertical offset from back argos arm to Front Argos Arm pivot on shooter
% l_10: horizontal offset for top roller of intake
% l_11: vertical offset for top roller of intake

% Calculate top front position
% Calculate the intersection between two circles of radius R and r
% where R is centered at (0,0), and r is centered at (d,0)
% x = (d^2-r^2+R^2)/(2*d)
% y = sqrt(R^2-x^2)
R = Ball_Screw_Length;
r = l_5;
d = sqrt(l_2^2+l_4^2);
x = (d^2-r^2+R^2)/(2*d);
sqrt_input = R^2-x^2;
if sqrt_input >= 0
    y = sqrt(sqrt_input);
else
    y = 0;
end

% Calculate angle between lower front pivot and lower ball screw pivot
alpha = atan(-l_2/l_4);

% Use a rotation matrix to move (x,y) to intersection of ball screw at front arm
cos_alpha = cos(alpha);
sin_alpha = sin(alpha);
intersection_x = l_3 + x*cos_alpha - y*sin_alpha;
intersection_y = l_2 + x*sin_alpha + y*cos_alpha;

% Calculate top front position
Top_Front_Pivot_x = (intersection_x-l_3-l_4)*(Front_AA_Length/l_5)+l_3+l_4;
Top_Front_Pivot_y = intersection_y*(Front_AA_Length/l_5);

% Calculate the intersection between two circles of radius R and r
% where R is centered at (0,0), and r is centered at (d,0)
% x = (d^2-r^2+R^2)/(2*d)
% y = sqrt(R^2-x^2)
R = Back_AA_Length;
r = sqrt(l_8^2+l_9^2);  % distance between top front pivot and top back pivot
d = sqrt(Top_Front_Pivot_x^2+(Top_Front_Pivot_y-l_1)^2);
x = (d^2-r^2+R^2)/(2*d);
sqrt_input = R^2-x^2;
if sqrt_input >= 0
    y = sqrt(sqrt_input);
else
    y = 0;
end

% Calculate angle between lower back pivot and top front pivot
% The origin x is the same as lower back position
% The origin y is below the lower back position by distance l_1
alpha = atan((Top_Front_Pivot_y-l_1)/Top_Front_Pivot_x);

% Use a rotation matrix to move (x,y) to the top back pivot
cos_alpha = cos(alpha);
sin_alpha = sin(alpha);
Top_Back_Pivot_x = x*cos_alpha - y*sin_alpha;
Top_Back_Pivot_y = x*sin_alpha + y*cos_alpha + l_1;

% Calculate the shooter angle
Angle = atan((Top_Front_Pivot_y-Top_Back_Pivot_y)/(Top_Front_Pivot_x-Top_Back_Pivot_x)) - atan(l_9/l_8);
cos_Angle = cos(Angle);
sin_Angle = sin(Angle);

% Calculate the shooter height
Height = Top_Back_Pivot_y - l_6*sin_Angle - l_7*cos_Angle;

% Calculate the shooter gap to intake
Gap = sqrt((Top_Back_Pivot_x - l_10 - l_6*cos_Angle + l_7*sin_Angle)^2 + (Height-l_11)^2);

== matlab function Shooter_Arm_Controls/Get_Arm_Lengths ==
  data: Angle input; Height input; Gap input; l_1 input; l_2 input; l_3 input; l_4 input; l_5 input; l_6 input; l_7 input; l_8 input; l_9 input; Back_AA_Length output; l_10 input; l_11 input; Front_AA_Length output; Ball_Screw_Length output
function [Back_AA_Length,Front_AA_Length,Ball_Screw_Length] = Get_Arm_Lengths(Angle, Height, Gap,l_1,l_2,l_3,l_4,l_5,l_6,l_7,l_8,l_9,l_10,l_11)

% Kinematic lengths
% l_1: vertical offset of back Argos Arm
% l_2: vertical offset of Ball Screw
% l_3: horizontal length from back argos arm to Ball Screw
% l_4: horizontal length from ball screw to front Argos Arm
% l_5: length from pivot of front argos arm to pivot of ball screw on that arm
% l_6: horizontal offset from the end of gap to Back Argos Arm pivot on shooter
% l_7: vertical offset from the end of gap to Back Argos Arm pivot on shooter
% l_8: horizontal offset from back argos arm to Front Argos Arm pivot on shooter
% l_9: vertical offset from back argos arm to Front Argos Arm pivot on shooter
% l_10: horizontal offset for top roller of intake
% l_11: vertical offset for top roller of intake

rot_cos = cos(Angle);
rot_sin = sin(Angle);
Rot_Mat = [ rot_cos, -rot_sin;...
            rot_sin, rot_cos ];

% Top back pivot
sqrt_input = Gap^2 - (Height - l_11 )^2;
if sqrt_input >= 0
    Top_Back_Pivot = [l_10 + sqrt(sqrt_input); Height] + mtimes(Rot_Mat, [l_6; l_7]);
else
    Top_Back_Pivot = [l_10; Height] + mtimes(Rot_Mat, [l_6; l_7]);
end

% Back Argos Arm Straight Length
Back_AA_Length = sqrt((Top_Back_Pivot(1,1))^2 + (Top_Back_Pivot(2,1)- l_1 )^2);

% Top front pivot
Top_Front_Pivot = Top_Back_Pivot + Rot_Mat*[l_8 ; l_9 ];

% Front Argos Arm Straight Length
Front_AA_Length = sqrt((Top_Front_Pivot(1,1)-(l_3 + l_4 ))^2 + Top_Front_Pivot(2,1)^2);

% Ball Screw Straight Length
Ball_Screw_Length = sqrt((l_4 - (l_3+l_4-Top_Front_Pivot(1,1))*(l_5/Front_AA_Length))^2 + ((Top_Front_Pivot(2,1)*(l_5/Front_AA_Length)-l_2))^2);

end

== matlab function Shooter_Arm_Controls/Back_AA_To_Extentions ==
  data: Top_Ext_Dist output; Bottom_Ext_Dist output; Straight_Line_Dist input; AA_spacing input; AA_Length input; Bot_Min_Ext input; Bot_Max_Ext input; Top_Min_Ext input; Top_Max_Ext input; Bottom_Fast_RL_Range output
function [Top_Ext_Dist,Bottom_Ext_Dist,Bottom_Fast_RL_Range] = Back_AA_To_Extentions(Straight_Line_Dist,AA_spacing,AA_Length,Bot_Min_Ext,Bot_Max_Ext,Top_Min_Ext,Top_Max_Ext)

% Total linear extension needed from top and bottom arms
E = sqrt(Straight_Line_Dist^2 - AA_spacing^2) - AA_Length;

Bottom_First_Ext = 90+25;
Split_Factor = 0.32;

if E <= Bot_Min_Ext + Top_Min_Ext;
    % both at minimum
    Bottom_Ext_Dist = Bot_Min_Ext;
    Top_Ext_Dist = Top_Min_Ext;
elseif E <= Bottom_First_Ext + Top_Min_Ext + Bot_Min_Ext
    % raise bottom a certain distance before top
    Bottom_Ext_Dist = E - Top_Min_Ext;
    Top_Ext_Dist = Top_Min_Ext;
else
    % raise bottom and top together
    E_remaining = E - Bottom_First_Ext - Top_Min_Ext - Bot_Min_Ext;
    Bottom_Ext_Dist = min(max(Bottom_First_Ext+Bot_Min_Ext+E_remaining*Split_Factor,Bot_Min_Ext),Bot_Max_Ext);
    Top_Ext_Dist = min(max(E-Bottom_Ext_Dist,Top_Min_Ext),Top_Max_Ext);
end

Bottom_Fast_RL_Range = Bot_Min_Ext + Bottom_First_Ext;

end
